simulink model "rp_ofc_lin"  (R2023b)
settings: Solver=ode45  StartTime=0.0  StopTime=rp_p.simtime  RelTol=1e-6  AbsTol=1e-6
values from neighbouring files (symbols this model uses):
  rp_p = rp_parameters()    [rp_mainfile_modelling_comparison_a.m]    (also in rp_mainfile_ofc_comparison_b.m)
undefined symbols (not defined in the file or in its folder): rp_lin_model, rp_observer
settings Model: Creator=cgorman  LastModifiedBy=cgorman

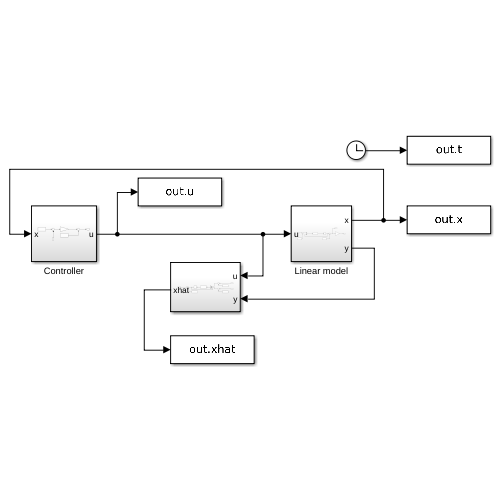
[thumbnail: Simulink's stored preview of the top-level diagram]
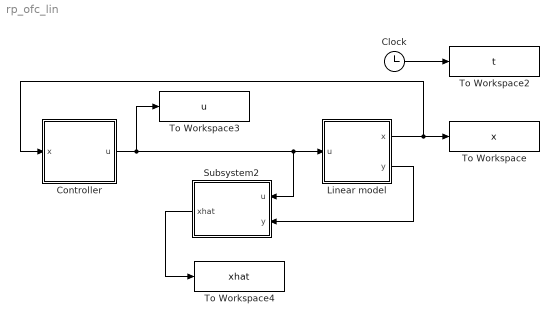
== system rp_ofc_lin ==
  Clock : Clock
  Controller : Subsystem
  Linear model : Subsystem
  Subsystem2 : Subsystem
  To Workspace : ToWorkspace  VariableName=x  SampleTime=-1
  To Workspace2 : ToWorkspace  VariableName=t  SampleTime=-1
  To Workspace3 : ToWorkspace  VariableName=u
  To Workspace4 : ToWorkspace  VariableName=xhat
  wires:
  Controller/1(u) -> Linear model/1(u), Subsystem2/1(u), To Workspace3/1
  Linear model/1(x) -> Controller/1(x), To Workspace/1
  Linear model/2(y) -> Subsystem2/2(y)
  Clock/1 -> To Workspace2/1
  Subsystem2/1(xhat) -> To Workspace4/1

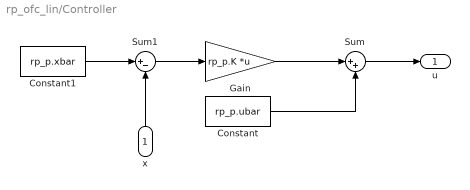
== system rp_ofc_lin/Controller ==
  x : Inport
  Constant : Constant  Value=rp_p.ubar
  Constant1 : Constant  Value=rp_p.xbar
  Gain : Gain  Gain=rp_p.K  Multiplication=Matrix(K*u)
  Sum : Sum  Inputs=|++
  Sum1 : Sum  Inputs=|+-
  u : Outport
  wires:
  Constant/1 -> Sum/2
  Gain/1 -> Sum/1
  Constant1/1 -> Sum1/1
  x/1 -> Sum1/2
  Sum1/1 -> Gain/1
  Sum/1 -> u/1

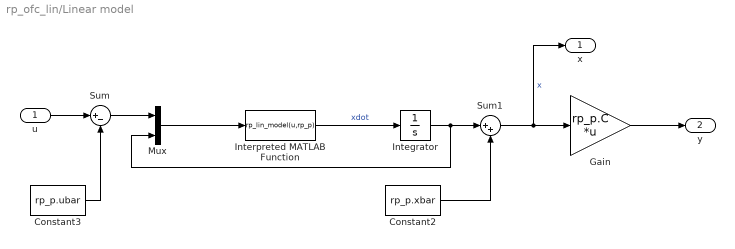
== system rp_ofc_lin/Linear model ==
  u : Inport
  Constant2 : Constant  Value=rp_p.xbar
  Constant3 : Constant  Value=rp_p.ubar
  Gain : Gain  Gain=rp_p.C  Multiplication=Matrix(K*u)
  Integrator : Integrator  InitialCondition=rp_p.iclin
  Interpreted MATLAB Function : MATLABFcn  MATLABFcn=rp_lin_model(u,rp_p)
  Mux : Mux  Inputs=2
  Sum : Sum  Inputs=|+-
  Sum1 : Sum  Inputs=|++
  x : Outport
  y : Outport  Port=2
  wires:
  Sum/1 -> Mux/1
  u/1 -> Sum/1
  Mux/1 -> Interpreted MATLAB Function/1
  Constant2/1 -> Sum1/2
  Constant3/1 -> Sum/2
  Interpreted MATLAB Function/1 -> Integrator/1  "xdot"
  Integrator/1 -> Mux/2, Sum1/1
  Sum1/1 -> Gain/1, x/1  "x"
  Gain/1 -> y/1

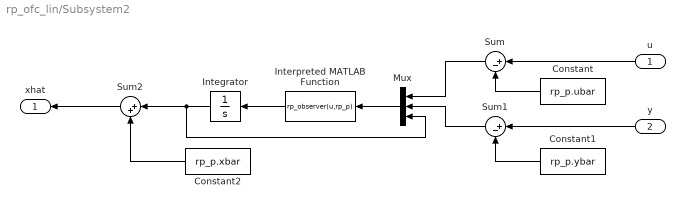
== system rp_ofc_lin/Subsystem2 ==
  u : Inport
  y : Inport  Port=2
  Constant : Constant  Value=rp_p.ubar
  Constant1 : Constant  Value=rp_p.ybar
  Constant2 : Constant  Value=rp_p.xbar
  Integrator : Integrator  InitialCondition=rp_p.icobs
  Interpreted MATLAB Function : MATLABFcn  MATLABFcn=rp_observer(u,rp_p)
  Mux : Mux  Inputs=3
  Sum : Sum  Inputs=|+-
  Sum1 : Sum  Inputs=|+-
  Sum2 : Sum  Inputs=|++
  xhat : Outport
  wires:
  Mux/1 -> Interpreted MATLAB Function/1
  Sum1/1 -> Mux/2
  Constant2/1 -> Sum2/2
  Sum2/1 -> xhat/1
  Sum/1 -> Mux/1
  Constant/1 -> Sum/2
  Integrator/1 -> Sum2/1, Mux/3
  y/1 -> Sum1/1
  Interpreted MATLAB Function/1 -> Integrator/1
  Constant1/1 -> Sum1/2
  u/1 -> Sum/1
